simulink model "BallInTube_simulation_nonlinear"  (R2024b)
settings: Solver=VariableStepAuto  StartTime=0.0  StopTime=50  RelTol=1e-3
undefined symbols (not defined in the file): a1, a2, a3, initial, k_w, Kd, Ki, Kp, lower_sat, tau_w, upper_sat
libraries: simulink x1, slpidlib x1
settings Model: Creator=elias  LastModifiedBy=elias

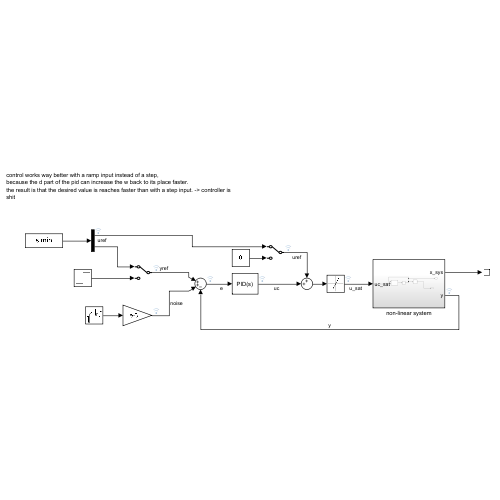
[thumbnail: Simulink's stored preview of the top-level diagram]
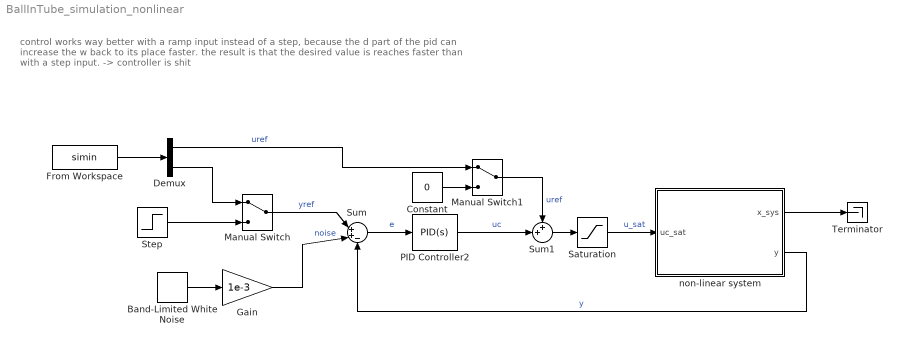
== system BallInTube_simulation_nonlinear ==
  note: control works way better with a ramp input instead of a step,
      | because the d part of the pid can increase the w back to its place faster.
      | the result is that the desired value is reaches faster than with a step input. -> controller is shit
  Band-Limited White Noise : simulink/Sources/Band-Limited White Noise  Cov=[0.1]  Ts=0.1  seed=[23341]
  Constant : Constant  Value=0
  Demux : Demux  Outputs=2
  From Workspace : FromWorkspace  VariableName=simin
  Gain : Gain  Gain=1e-3
  Manual Switch : ManualSwitch
  Manual Switch1 : ManualSwitch
  PID Controller2 : slpidlib/PID Controller  Controller=PID  Form=Parallel  TimeDomain=Continuous-time  UseExternalTs=off  SampleTime=-1  IntegratorMethod=Forward Euler  FilterMethod=Forward Euler  ControllerParametersSource=internal  P=Kp  I=Ki  UseKiTs=off  D=Kd  UseExternalDerivativeSource=off  N=100  UseFilter=on  TunerSelectOption=Transfer Function Based (PID Tuner App)  InitialConditionSource=internal  InitialConditionForIntegrator=0  InitialConditionForFilter=0  DifferentiatorICPrevScaledInput=0  ExternalReset=none  TrackingMode=off  Kt=1  LimitOutput=off  SatLimitsSource=internal  UpperSaturationLimit=inf  LowerSaturationLimit=-inf  LinearizeAsGain=on  AntiWindupMode=none  Kb=1  LimitIntegrator=off  UpperIntegratorSaturationLimit=inf  LowerIntegratorSaturationLimit=-inf  POutMin=[]  POutMax=[]  IOutMin=[]  IOutMax=[]  DOutMin=[]  DOutMax=[]  NOutMin=[]  NOutMax=[]  SumOutMin=[]  SumOutMax=[]  SaturationOutMin=[]  SaturationOutMax=[]  PParamMin=[]  PParamMax=[]  IParamMin=[]  IParamMax=[]  DParamMin=[]  DParamMax=[]  NParamMin=[]  NParamMax=[]  KbParamMin=[]  KbParamMax=[]  KtParamMin=[]  KtParamMax=[]  KbOutMin=[]  KbOutMax=[]  KtOutMin=[]  KtOutMax=[]  IntegratorOutMin=[]  IntegratorOutMax=[]  FilterOutMin=[]  FilterOutMax=[]  SumI1OutMin=[]  SumI1OutMax=[]  SumI2OutMin=[]  SumI2OutMax=[]  SumI3OutMin=[]  SumI3OutMax=[]  SumI4OutMin=[]  SumI4OutMax=[]  SumDOutMin=[]  SumDOutMax=[]  DifferentiatorOutMin=[]  DifferentiatorOutMax=[]  FilterDiffOutCoefMin=[]  FilterDiffOutCoefMax=[]  ReciprocalOutMin=[]  ReciprocalOutMax=[]  SumDenOutMin=[]  SumDenOutMax=[]  SumNumOutMin=[]  SumNumOutMax=[]  DivideOutMin=[]  DivideOutMax=[]  UdiffTsProdOutMin=[]  UdiffTsProdOutMax=[]  NTsProdOutMin=[]  NTsProdOutMax=[]  UintegralTsProdOutMin=[]  UintegralTsProdOutMax=[]  UngainTsProdOutMin=[]  UngainTsProdOutMax=[]  ClampingZeroOutDataTypeStr=Inherit: Inherit via back propagation  ClampingZeroOutMin=[]  ClampingZeroOutMax=[]  FilterDenConstantOutDataTypeStr=Inherit: Inherit via back propagation  FilterDenConstantOutMin=[]  FilterDenConstantOutMax=[]  PCopyOutDataTypeStr=Inherit: Inherit via back propagation  PCopyOutMin=[]  PCopyOutMax=[]  NCopyOutDataTypeStr=Inherit: Inherit via back propagation  NCopyOutMin=[]  NCopyOutMax=[]  IntegratorContinuousStateAttributes=''  IntegratorStateMustResolveToSignalObject=off  IntegratorRTWStateStorageClass=Auto  FilterContinuousStateAttributes=''  FilterStateMustResolveToSignalObject=off  FilterRTWStateStorageClass=Auto  ParallelPVariant=InternalParameters  IdealPVariant=Disabled  IVariant=InternalParameters  DVariant=InternalParameters  IntegratorVariant=Continuous  SatVariant=Disabled  AWVariant=Passthrough  PCopyVariant=Disabled  TRVariant=Disabled  FdbkBlocksVariant=Forward  IdealPFdbkVariant=Disabled  SatFdbkVariant=Disabled  DerivativeFilterVariant=ContFilter  NVariant=InternalParameters  NCopyVariant=Disabled  FilterICVariant=InternalICsFilter  IntegratorICVariant=InternalICs  ExternalResetVariant=Disabled  TRSumVariant=Passthrough  SumFdbkVariant=Disabled  SumVariant=Sum_PID  TsampFilterVariant=InternalTs  TsampNgainVariant=Passthrough  TsampIntegralVariant=Disabled_SignalSpec  ExternalSaturationOutDataTypeStr=Inherit: Same as second input  DerivativeSourceVariant=ErrorSignal  PreIntVariant=InternalPreInt
  Saturation : Saturate  UpperLimit=5  LowerLimit=0
  Step : Step  SampleTime=0
  Sum : Sum  Inputs=|++-
  Sum1 : Sum  Inputs=++|
  Terminator : Terminator
  non-linear system : Subsystem
  wires:
  Sum/1 -> PID Controller2/1  "e"
  PID Controller2/1 -> Sum1/2  "uc"
  non-linear system/2(y) -> Sum/3  "y"
  Saturation/1 -> non-linear system/1(uc_sat)  "u_sat"
  non-linear system/1(x_sys) -> Terminator/1
  Band-Limited White Noise/1 -> Gain/1
  Gain/1 -> Sum/2  "noise"
  From Workspace/1 -> Demux/1
  Manual Switch/1 -> Sum/1  "yref"
  Manual Switch1/1 -> Sum1/1  "uref"
  Demux/2 -> Manual Switch/1
  Demux/1 -> Manual Switch1/1  "uref"
  Constant/1 -> Manual Switch1/2
  Step/1 -> Manual Switch/2
  Sum1/1 -> Saturation/1

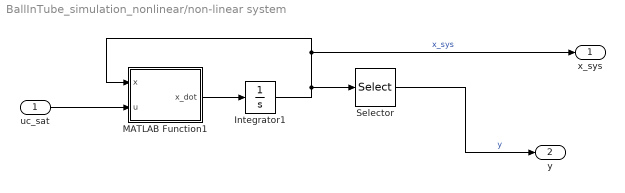
== system BallInTube_simulation_nonlinear/non-linear system ==
  uc_sat : Inport
  Integrator1 : Integrator  InitialCondition=initial  LimitOutput=on  UpperSaturationLimit=upper_sat  LowerSaturationLimit=lower_sat
  MATLAB Function1 : MATLAB Function  TreatAsAtomicUnit=on
  Selector : Selector  InputPortWidth=3  IndexOptions=Index vector (dialog)  Indices=1  OutputSizes=1
  x_sys : Outport
  y : Outport  Port=2
  wires:
  Integrator1/1 -> Selector/1, MATLAB Function1/1(x), x_sys/1  "x_sys"
  MATLAB Function1/1(x_dot) -> Integrator1/1
  uc_sat/1 -> MATLAB Function1/2(u)
  Selector/1 -> y/1  "y"

== matlab function BallInTube_simulation_nonlinear/non-linear system/MATLAB Function1 ==
  data: x input; u input; x_dot output; a1 parameter; a2 parameter; a3 parameter; tau_w parameter; k_w parameter
function x_dot  = fcn(x,u,a1, a2, a3, tau_w, k_w)



%nonlinear set of equation
x_dot = [x(2); (a1*x(3)-a2*x(2))^2-a3; -x(3)/tau_w]+[0; 0; k_w/tau_w]*u;
